simulink model "comprobacion_de_sistema_lineal"  (R2023b)
settings: Solver=VariableStepAuto  StartTime=0.0  StopTime=10.0  RelTol=1e-3
libraries: simulink x2
settings Model: Creator=delga  LastModifiedBy=albsa

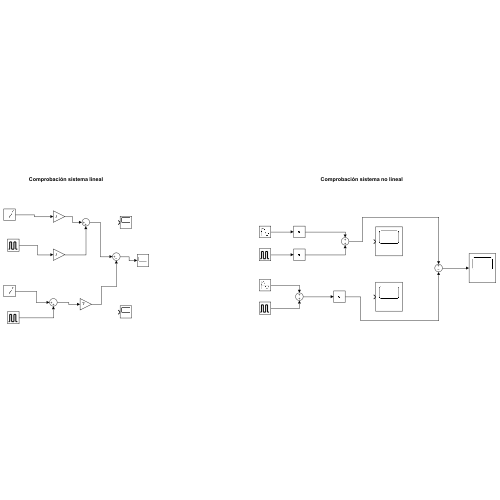
[thumbnail: Simulink's stored preview of the top-level diagram]
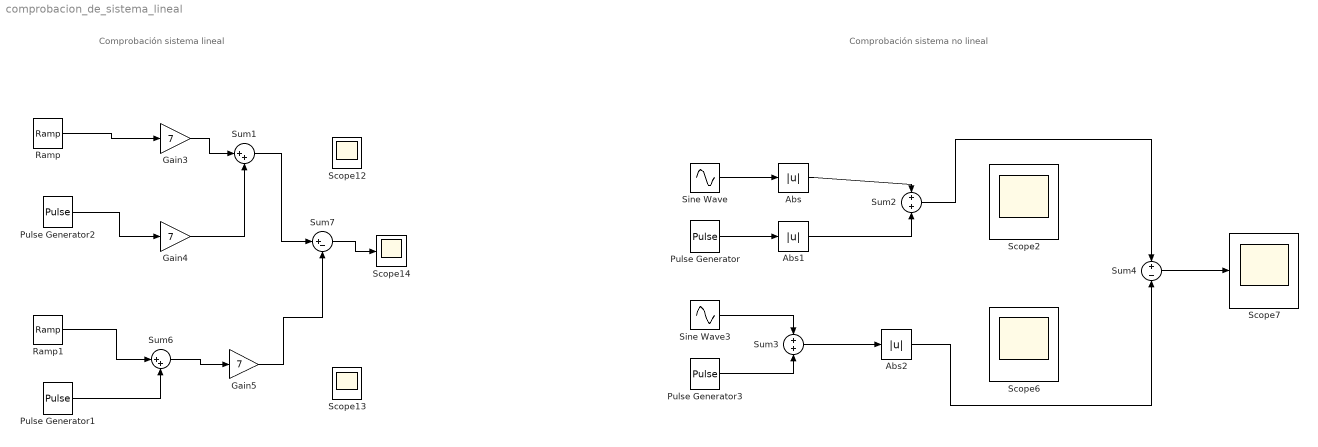
== system comprobacion_de_sistema_lineal ==
  note: Comprobación sistema lineal
  note: Comprobación sistema no lineal
  Abs : Abs  SaturateOnIntegerOverflow=off
  Abs1 : Abs  SaturateOnIntegerOverflow=off
  Abs2 : Abs  SaturateOnIntegerOverflow=off
  Gain3 : Gain  Gain=7
  Gain4 : Gain  Gain=7
  Gain5 : Gain  Gain=7
  Pulse Generator : DiscretePulseGenerator  PulseType=Time based  Period=10  PulseWidth=5
  Pulse Generator1 : DiscretePulseGenerator  PulseType=Time based  Period=10
  Pulse Generator2 : DiscretePulseGenerator  PulseType=Time based  Period=10
  Pulse Generator3 : DiscretePulseGenerator  PulseType=Time based  Period=10  PulseWidth=5
  Ramp : simulink/Sources/Ramp  slope=1  start=0  InitialOutput=0
  Ramp1 : simulink/Sources/Ramp  slope=1  start=0  InitialOutput=0
  Scope{2,6..7,12..14} (6 alike) : Scope
  Sine Wave : Sin  Amplitude=2  SampleTime=0
  Sine Wave3 : Sin  Amplitude=2  SampleTime=0
  Sum1 : Sum  Inputs=|++
  Sum2 : Sum
  Sum3 : Sum
  Sum4 : Sum  Inputs=+-
  Sum6 : Sum  Inputs=|++
  Sum7 : Sum  Inputs=|+-  RndMeth=Round
  wires:
  Sum6/1 -> Gain5/1
  Gain5/1 -> Sum7/2
  Gain4/1 -> Sum1/2
  Sum7/1 -> Scope14/1
  Ramp/1 -> Gain3/1
  Sum1/1 -> Sum7/1
  Ramp1/1 -> Sum6/1
  Pulse Generator1/1 -> Sum6/2
  Gain3/1 -> Sum1/1
  Pulse Generator2/1 -> Gain4/1
  Sum4/1 -> Scope7/1
  Abs2/1 -> Sum4/2
  Pulse Generator3/1 -> Sum3/2
  Sum2/1 -> Sum4/1
  Sine Wave3/1 -> Sum3/1
  Pulse Generator/1 -> Abs1/1
  Abs1/1 -> Sum2/2
  Sum3/1 -> Abs2/1
  Abs/1 -> Sum2/1
  Sine Wave/1 -> Abs/1
